simulink model "assignment1_aai"  (R2022b)
settings: Solver=FixedStepAuto  StartTime=0.0  StopTime=10.0  FixedStep=1e-3  RelTol=1e-3  EnableMultiTasking=on
undefined symbols (not defined in the file): D0, D10, D11, D12, D2, D4, D5, D7, D8, D9, PTA0, PTA2, PTB23, PTB9, PTC16, PTC3, PTC4, PTD0, PTD2, PTD3
libraries: frdmk64flib x10
settings Model: ExtModeTrigDuration=5  Creator=samiaanwar  LastModifiedBy=tammyz
settings OptimizationCC: EnhancedBackFolding=on  PassReuseOutputArgsAs=Individual arguments  ZeroExternalMemoryAtStartup=off  ZeroInternalMemoryAtStartup=off  MaxStackSize=64  OptimizeBlockOrder=speed  DifferentSizesBufferReuse=on  OptimizationCustomize=off  EfficientTunableParamExpr=on
settings DebuggingCC: ParameterTunabilityLossMsg=error
settings HardwareCC: ProdBitPerPointer=32  ProdBitPerSizeT=32  ProdBitPerPtrDiffT=32  ProdLargestAtomicInteger=Long  ProdLargestAtomicFloat=Double  ProdWordSize=32  ProdHWDeviceType=ARM Compatible->ARM Cortex
settings SFSimCC: MATLABDynamicMemAlloc=off
settings RTWCC: Description=Embedded Coder  SystemTargetFile=ert.tlc  HardwareBoard=NXP FRDM-K64F  TLCOptions="-aInlineSetEventsForThisBaseRateFcn=TLC_FALSE -aSuppressMultiTaskScheduler=TLC_FALSE  -aRateBasedStepFcn=0"  TemplateMakefile=ert_default_tmf  Toolchain=GNU Tools for ARM Embedded Processors
settings CodeAppCC: ForceParamTrailComments=on  IgnoreCustomStorageClasses=off  OperatorAnnotations=on  SimulinkDataObjDesc=on  SFDataObjDesc=on  InsertBlockDesc=on
settings ERTTargetCC: ExtModeTransport=4  ExtModeMexFile=sendToCommService

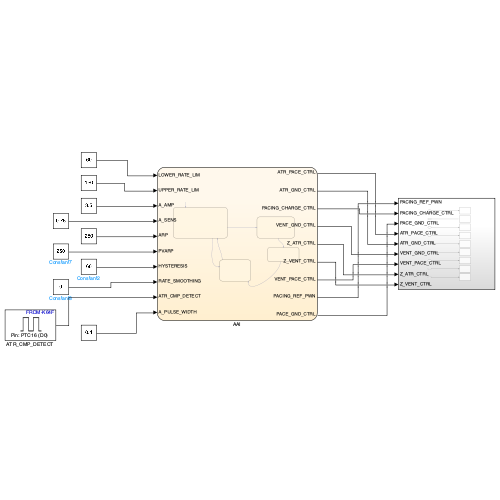
[thumbnail: Simulink's stored preview of the top-level diagram]
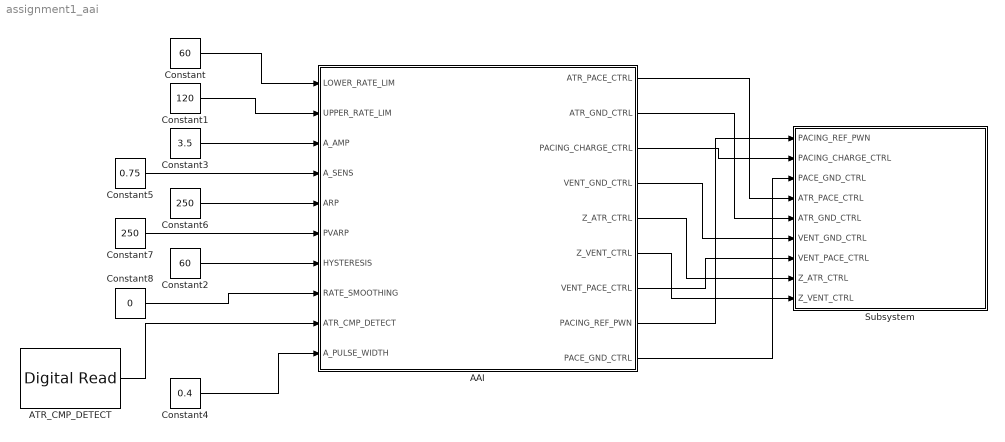
== system assignment1_aai ==
  AAI : Stateflow chart  TreatAsAtomicUnit=on
  ATR_CMP_DETECT : frdmk64flib/Digital Read  Whichpin=PTC16 (D0)  SampleTime=-1
  Constant : Constant  Value=60
  Constant1 : Constant  Value=120
  Constant2 : Constant  Value=60
  Constant3 : Constant  Value=3.5
  Constant4 : Constant  Value=0.4
  Constant5 : Constant  Value=0.75
  Constant6 : Constant  Value=250
  Constant7 : Constant  Value=250
  Constant8 : Constant  Value=0
  Subsystem : Subsystem
  wires:
  ATR_CMP_DETECT/1 -> AAI/9(ATR_CMP_DETECT)
  Constant/1 -> AAI/1(LOWER_RATE_LIM)
  Constant1/1 -> AAI/2(UPPER_RATE_LIM)
  Constant2/1 -> AAI/7(HYSTERESIS)
  Constant3/1 -> AAI/3(A_AMP)
  Constant4/1 -> AAI/10(A_PULSE_WIDTH)
  AAI/1(ATR_PACE_CTRL) -> Subsystem/4(ATR_PACE_CTRL)
  AAI/2(ATR_GND_CTRL) -> Subsystem/5(ATR_GND_CTRL)
  AAI/3(PACING_CHARGE_CTRL) -> Subsystem/2(PACING_CHARGE_CTRL)
  Constant5/1 -> AAI/4(A_SENS)
  Constant6/1 -> AAI/5(ARP)
  Constant7/1 -> AAI/6(PVARP)
  Constant8/1 -> AAI/8(RATE_SMOOTHING)
  AAI/4(VENT_GND_CTRL) -> Subsystem/6(VENT_GND_CTRL)
  AAI/5(Z_ATR_CTRL) -> Subsystem/8(Z_ATR_CTRL)
  AAI/6(Z_VENT_CTRL) -> Subsystem/9(Z_VENT_CTRL)
  AAI/7(VENT_PACE_CTRL) -> Subsystem/7(VENT_PACE_CTRL)
  AAI/8(PACING_REF_PWN) -> Subsystem/1(PACING_REF_PWN)
  AAI/9(PACE_GND_CTRL) -> Subsystem/3(PACE_GND_CTRL)

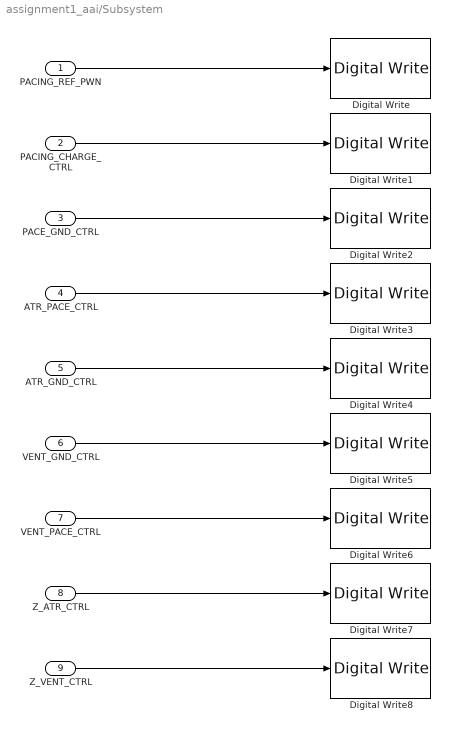
== system assignment1_aai/Subsystem ==
  PACING_REF_PWN : Inport
  PACING_CHARGE_CTRL : Inport  Port=2
  PACE_GND_CTRL : Inport  Port=3
  ATR_PACE_CTRL : Inport  Port=4
  ATR_GND_CTRL : Inport  Port=5
  VENT_GND_CTRL : Inport  Port=6
  VENT_PACE_CTRL : Inport  Port=7
  Z_ATR_CTRL : Inport  Port=8
  Z_VENT_CTRL : Inport  Port=9
  Digital Write : frdmk64flib/Digital Write  Whichpin=PTA2 (D5)
  Digital Write1 : frdmk64flib/Digital Write  Whichpin=PTB9 (D2)
  Digital Write2 : frdmk64flib/Digital Write  Whichpin=PTD0 (D10)
  Digital Write3 : frdmk64flib/Digital Write  Whichpin=PTA0 (D8)
  Digital Write4 : frdmk64flib/Digital Write  Whichpin=PTD2 (D11)
  Digital Write5 : frdmk64flib/Digital Write  Whichpin=PTD3 (D12)
  Digital Write6 : frdmk64flib/Digital Write  Whichpin=PTC4 (D9)
  Digital Write7 : frdmk64flib/Digital Write  Whichpin=PTB23 (D4)
  Digital Write8 : frdmk64flib/Digital Write  Whichpin=PTC3 (D7)
  wires:
  PACING_REF_PWN/1 -> Digital Write/1
  PACING_CHARGE_CTRL/1 -> Digital Write1/1
  PACE_GND_CTRL/1 -> Digital Write2/1
  ATR_PACE_CTRL/1 -> Digital Write3/1
  ATR_GND_CTRL/1 -> Digital Write4/1
  VENT_GND_CTRL/1 -> Digital Write5/1
  VENT_PACE_CTRL/1 -> Digital Write6/1
  Z_ATR_CTRL/1 -> Digital Write7/1
  Z_VENT_CTRL/1 -> Digital Write8/1

== stateflow chart assignment1_aai/AAI ==
  state CHARGING_C22
    ATR_PACE_CTRL = false
    ATR_GND_CTRL = true
    PACING_CHARGE_CTRL = true
    PACING_REF_PWN = A_AMP/5
    PACE_GND_CTRL = true
    VENT_PACE_CTRL = false
    VENT_GND_CTRL = false
    Z_ATR_CTRL = false
    Z_VENT_CTRL = false
  state DISCHARGING
    PACING_CHARGE_CTRL = false
    PACE_GND_CTRL = true
    ATR_GND_CTRL = false
  state INTERMEDIATE
    ATR_PACE_CTRL = true
  state REFRACTORY
    entry:
    ATR_PACE_CTRL = false
    ATR_GND_CTRL = true
  (default) -> CHARGING_C22
  CHARGING_C22 -> DISCHARGING [order 2]
  CHARGING_C22 -> REFRACTORY [order 1] : [ATR_CMP_DETECT]
  REFRACTORY -> CHARGING_C22 : after(ARP, msec)
  DISCHARGING -> INTERMEDIATE
  INTERMEDIATE -> REFRACTORY : after(A_PULSE_WIDTH, msec)
  data: LOWER_RATE_LIM input double; UPPER_RATE_LIM input double; A_AMP input double; A_SENS input double; ARP input double; PVARP input double; HYSTERESIS input double; RATE_SMOOTHING input double; ATR_CMP_DETECT input; ATR_PACE_CTRL output; ATR_GND_CTRL output; PACING_CHARGE_CTRL output; A_PULSE_WIDTH input; VENT_GND_CTRL output; Z_ATR_CTRL output; Z_VENT_CTRL output; VENT_PACE_CTRL output; PACING_REF_PWN output; PACE_GND_CTRL output
